simulink model "EPA_Walker"  (R2018a)
settings: Solver=FixedStepDiscrete  StartTime=0.0  StopTime=inf  FixedStep=0.001  RelTol=1e-3  EnableMultiTasking=on
model workspace (MAT data in the model file):
  MCOS : class17 (value not decoded)
undefined symbols (not defined in the file or in its folder): bits_current, bits_GRF, bits_Kd, bits_Kp, bits_position, bits_velocity, deadzone_in_TIB, deadzone_out_TIB, GRF_MAX, GRF_MIN, k_p_TIB, KD_MAX, KD_MIN, KP_MAX, KP_MIN, P_MAX, P_MIN, PressureFilter_CutOffFreq, PressureFilter_Gain, ReadingVoltage, T_MAX, T_MIN, V_MAX, V_MIN, voltageBias_GAS, voltageBias_GL, voltageBias_HAM, voltageBias_IL, voltageBias_POP, voltageBias_RF, voltageBias_SOL, voltageBias_TIB, voltageBias_VAS, voltageMultiplier_GAS, voltageMultiplier_GL, voltageMultiplier_HAM, voltageMultiplier_IL, voltageMultiplier_POP, voltageMultiplier_RF, voltageMultiplier_SOL, voltageMultiplier_TIB, voltageMultiplier_VAS, VoltageResolution
libraries: xpcethercatlib x139, simulink x19, peGeneralControl x18, slrtlib x9
(part 2 of 5)

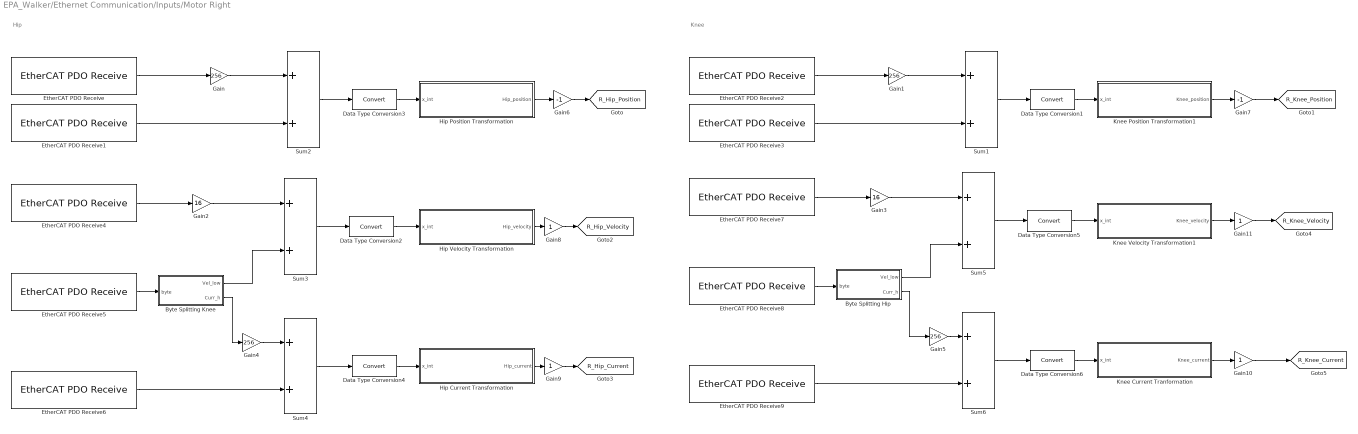
== system EPA_Walker/Ethernet Communication/Inputs/Motor Right ==
  note: Hip
  note: Knee
  Byte Splitting Hip : MATLAB Function  TreatAsAtomicUnit=on
  Byte Splitting Knee : MATLAB Function  TreatAsAtomicUnit=on
  Data Type Conversion{1..6} (6 alike) : DataTypeConversion
  EtherCAT PDO Receive : xpcethercatlib/EtherCAT PDO Receive  Priority=2  sig_name=Motors_R.Inputs.Byte0  sig_offset=256  sig_type=uint8  type_size=8  sig_dim=1  device_id=0  sample_time=0.001000
      settings: SourceProductName=Simulink Real-Time  SourceProductBaseCode=XP
  EtherCAT PDO Receive1 : xpcethercatlib/EtherCAT PDO Receive  Priority=2  sig_name=Motors_R.Inputs.Byte1  sig_offset=264  sig_type=uint8  type_size=8  sig_dim=1  device_id=0  sample_time=0.001000
      settings: SourceProductName=Simulink Real-Time  SourceProductBaseCode=XP
  EtherCAT PDO Receive2 : xpcethercatlib/EtherCAT PDO Receive  Priority=2  sig_name=Motors_R.Inputs.Byte5  sig_offset=296  sig_type=uint8  type_size=8  sig_dim=1  device_id=0  sample_time=0.001000
      settings: SourceProductName=Simulink Real-Time  SourceProductBaseCode=XP
  EtherCAT PDO Receive3 : xpcethercatlib/EtherCAT PDO Receive  Priority=2  sig_name=Motors_R.Inputs.Byte6  sig_offset=304  sig_type=uint8  type_size=8  sig_dim=1  device_id=0  sample_time=0.001000
      settings: SourceProductName=Simulink Real-Time  SourceProductBaseCode=XP
  EtherCAT PDO Receive4 : xpcethercatlib/EtherCAT PDO Receive  Priority=2  sig_name=Motors_R.Inputs.Byte2  sig_offset=272  sig_type=uint8  type_size=8  sig_dim=1  device_id=0  sample_time=0.001000
      settings: SourceProductName=Simulink Real-Time  SourceProductBaseCode=XP
  EtherCAT PDO Receive5 : xpcethercatlib/EtherCAT PDO Receive  Priority=2  sig_name=Motors_R.Inputs.Byte3  sig_offset=280  sig_type=uint8  type_size=8  sig_dim=1  device_id=0  sample_time=0.001000
      settings: SourceProductName=Simulink Real-Time  SourceProductBaseCode=XP
  EtherCAT PDO Receive6 : xpcethercatlib/EtherCAT PDO Receive  Priority=2  sig_name=Motors_R.Inputs.Byte4  sig_offset=288  sig_type=uint8  type_size=8  sig_dim=1  device_id=0  sample_time=0.001000
      settings: SourceProductName=Simulink Real-Time  SourceProductBaseCode=XP
  EtherCAT PDO Receive7 : xpcethercatlib/EtherCAT PDO Receive  Priority=2  sig_name=Motors_R.Inputs.Byte7  sig_offset=312  sig_type=uint8  type_size=8  sig_dim=1  device_id=0  sample_time=0.001000
      settings: SourceProductName=Simulink Real-Time  SourceProductBaseCode=XP
  EtherCAT PDO Receive8 : xpcethercatlib/EtherCAT PDO Receive  Priority=2  sig_name=Motors_R.Inputs.Byte8  sig_offset=320  sig_type=uint8  type_size=8  sig_dim=1  device_id=0  sample_time=0.001000
      settings: SourceProductName=Simulink Real-Time  SourceProductBaseCode=XP
  EtherCAT PDO Receive9 : xpcethercatlib/EtherCAT PDO Receive  Priority=2  sig_name=Motors_R.Inputs.Byte9  sig_offset=328  sig_type=uint8  type_size=8  sig_dim=1  device_id=0  sample_time=0.001000
      settings: SourceProductName=Simulink Real-Time  SourceProductBaseCode=XP
  Gain{,1,4..5} (4 alike) : Gain  Gain=256
  Gain{8..11} (4 alike) : Gain
  Gain2 : Gain  Gain=16
  Gain3 : Gain  Gain=16
  Gain6 : Gain  Gain=-1
  Gain7 : Gain  Gain=-1
  Hip Current Transformation : MATLAB Function  TreatAsAtomicUnit=on
  Hip Position Transformation : MATLAB Function  TreatAsAtomicUnit=on
  Hip Velocity Transformation : MATLAB Function  TreatAsAtomicUnit=on
  Knee Current Tranformation : MATLAB Function  TreatAsAtomicUnit=on
  Knee Position Transformation1 : MATLAB Function  TreatAsAtomicUnit=on
  Knee Velocity Transformation1 : MATLAB Function  TreatAsAtomicUnit=on
  Sum{1..6} (6 alike) : Sum
  tag scope: R_Hip_Current=global, R_Hip_Position=global, R_Hip_Velocity=global, R_Knee_Current=global, R_Knee_Position=global, R_Knee_Velocity=global
  wires:
  EtherCAT PDO Receive/1 -> Gain/1
  Sum2/1 -> Data Type Conversion3/1
  Data Type Conversion3/1 -> Hip Position Transformation/1(x_int)
  Gain/1 -> Sum2/1
  EtherCAT PDO Receive1/1 -> Sum2/2
  EtherCAT PDO Receive3/1 -> Sum1/2
  Gain1/1 -> Sum1/1
  Data Type Conversion1/1 -> Knee Position Transformation1/1(x_int)
  EtherCAT PDO Receive2/1 -> Gain1/1
  Sum1/1 -> Data Type Conversion1/1
  EtherCAT PDO Receive5/1 -> Byte Splitting Knee/1(byte)
  EtherCAT PDO Receive4/1 -> Gain2/1
  Gain2/1 -> Sum3/1
  Byte Splitting Knee/1(Vel_low) -> Sum3/2
  EtherCAT PDO Receive6/1 -> Sum4/2
  Data Type Conversion2/1 -> Hip Velocity Transformation/1(x_int)
  Sum3/1 -> Data Type Conversion2/1
  Data Type Conversion4/1 -> Hip Current Transformation/1(x_int)
  Sum4/1 -> Data Type Conversion4/1
  EtherCAT PDO Receive7/1 -> Gain3/1
  Sum5/1 -> Data Type Conversion5/1
  Gain3/1 -> Sum5/1
  EtherCAT PDO Receive9/1 -> Sum6/2
  EtherCAT PDO Receive8/1 -> Byte Splitting Hip/1(byte)
  Byte Splitting Hip/2(Curr_h) -> Gain5/1
  Sum6/1 -> Data Type Conversion6/1
  Byte Splitting Hip/1(Vel_low) -> Sum5/2
  Hip Position Transformation/1(Hip_position) -> Gain6/1
  Hip Velocity Transformation/1(Hip_velocity) -> Gain8/1
  Hip Current Transformation/1(Hip_current) -> Gain9/1
  Knee Position Transformation1/1(Knee_position) -> Gain7/1
  Knee Velocity Transformation1/1(Knee_velocity) -> Gain11/1
  Data Type Conversion5/1 -> Knee Velocity Transformation1/1(x_int)
  Knee Current Tranformation/1(Knee_current) -> Gain10/1
  Data Type Conversion6/1 -> Knee Current Tranformation/1(x_int)
  Gain4/1 -> Sum4/1
  Byte Splitting Knee/2(Curr_h) -> Gain4/1
  Gain5/1 -> Sum6/1
  Gain6/1 -> [R_Hip_Position]
  Gain7/1 -> [R_Knee_Position]
  Gain8/1 -> [R_Hip_Velocity]
  Gain9/1 -> [R_Hip_Current]
  Gain10/1 -> [R_Knee_Current]
  Gain11/1 -> [R_Knee_Velocity]

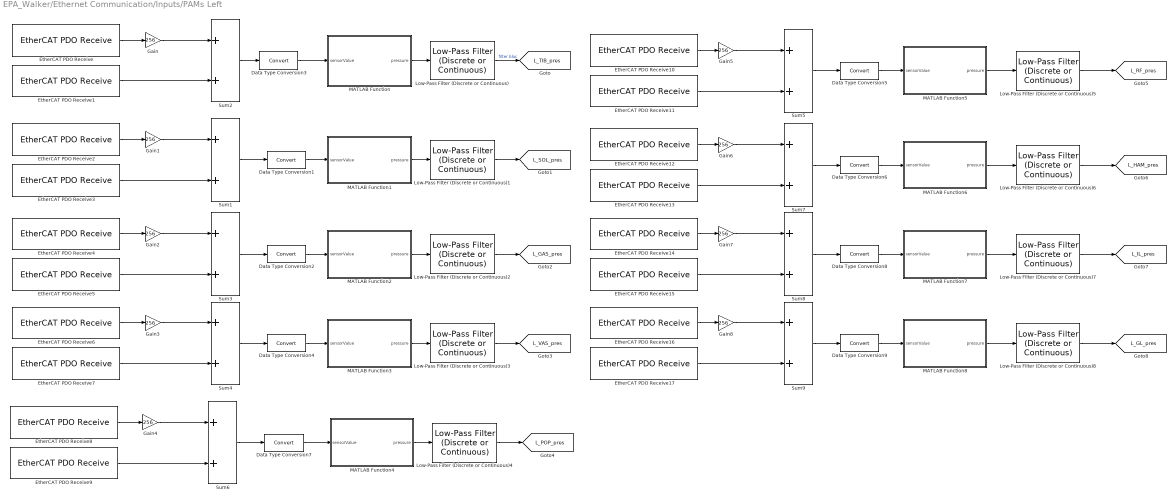
== system EPA_Walker/Ethernet Communication/Inputs/PAMs Left ==
  Data Type Conversion{1..9} (9 alike) : DataTypeConversion
  EtherCAT PDO Receive : xpcethercatlib/EtherCAT PDO Receive  Priority=2  sig_name=PAMs_L.Inputs.Byte0  sig_offset=1024  sig_type=uint8  type_size=8  sig_dim=1  device_id=0  sample_time=0.001000
      settings: SourceProductName=Simulink Real-Time  SourceProductBaseCode=XP
  EtherCAT PDO Receive1 : xpcethercatlib/EtherCAT PDO Receive  Priority=2  sig_name=PAMs_L.Inputs.Byte1  sig_offset=1032  sig_type=uint8  type_size=8  sig_dim=1  device_id=0  sample_time=0.001000
      settings: SourceProductName=Simulink Real-Time  SourceProductBaseCode=XP
  EtherCAT PDO Receive10 : xpcethercatlib/EtherCAT PDO Receive  Priority=2  sig_name=PAMs_L.Inputs.Byte10  sig_offset=1104  sig_type=uint8  type_size=8  sig_dim=1  device_id=0  sample_time=0.001000
      settings: SourceProductName=Simulink Real-Time  SourceProductBaseCode=XP
  EtherCAT PDO Receive11 : xpcethercatlib/EtherCAT PDO Receive  Priority=2  sig_name=PAMs_L.Inputs.Byte11  sig_offset=1112  sig_type=uint8  type_size=8  sig_dim=1  device_id=0  sample_time=0.001000
      settings: SourceProductName=Simulink Real-Time  SourceProductBaseCode=XP
  EtherCAT PDO Receive12 : xpcethercatlib/EtherCAT PDO Receive  Priority=2  sig_name=PAMs_L.Inputs.Byte12  sig_offset=1120  sig_type=uint8  type_size=8  sig_dim=1  device_id=0  sample_time=0.001000
      settings: SourceProductName=Simulink Real-Time  SourceProductBaseCode=XP
  EtherCAT PDO Receive13 : xpcethercatlib/EtherCAT PDO Receive  Priority=2  sig_name=PAMs_L.Inputs.Byte13  sig_offset=1128  sig_type=uint8  type_size=8  sig_dim=1  device_id=0  sample_time=0.001000
      settings: SourceProductName=Simulink Real-Time  SourceProductBaseCode=XP
  EtherCAT PDO Receive14 : xpcethercatlib/EtherCAT PDO Receive  Priority=2  sig_name=PAMs_L.Inputs.Byte14  sig_offset=1136  sig_type=uint8  type_size=8  sig_dim=1  device_id=0  sample_time=0.001000
      settings: SourceProductName=Simulink Real-Time  SourceProductBaseCode=XP
  EtherCAT PDO Receive15 : xpcethercatlib/EtherCAT PDO Receive  Priority=2  sig_name=PAMs_L.Inputs.Byte15  sig_offset=1144  sig_type=uint8  type_size=8  sig_dim=1  device_id=0  sample_time=0.001000
      settings: SourceProductName=Simulink Real-Time  SourceProductBaseCode=XP
  EtherCAT PDO Receive16 : xpcethercatlib/EtherCAT PDO Receive  Priority=2  sig_name=PAMs_L.Inputs.Byte16  sig_offset=1152  sig_type=uint8  type_size=8  sig_dim=1  device_id=0  sample_time=0.001000
      settings: SourceProductName=Simulink Real-Time  SourceProductBaseCode=XP
  EtherCAT PDO Receive17 : xpcethercatlib/EtherCAT PDO Receive  Priority=2  sig_name=PAMs_L.Inputs.Byte17  sig_offset=1160  sig_type=uint8  type_size=8  sig_dim=1  device_id=0  sample_time=0.001000
      settings: SourceProductName=Simulink Real-Time  SourceProductBaseCode=XP
  EtherCAT PDO Receive2 : xpcethercatlib/EtherCAT PDO Receive  Priority=2  sig_name=PAMs_L.Inputs.Byte2  sig_offset=1040  sig_type=uint8  type_size=8  sig_dim=1  device_id=0  sample_time=0.001000
      settings: SourceProductName=Simulink Real-Time  SourceProductBaseCode=XP
  EtherCAT PDO Receive3 : xpcethercatlib/EtherCAT PDO Receive  Priority=2  sig_name=PAMs_L.Inputs.Byte3  sig_offset=1048  sig_type=uint8  type_size=8  sig_dim=1  device_id=0  sample_time=0.001000
      settings: SourceProductName=Simulink Real-Time  SourceProductBaseCode=XP
  EtherCAT PDO Receive4 : xpcethercatlib/EtherCAT PDO Receive  Priority=2  sig_name=PAMs_L.Inputs.Byte4  sig_offset=1056  sig_type=uint8  type_size=8  sig_dim=1  device_id=0  sample_time=0.001000
      settings: SourceProductName=Simulink Real-Time  SourceProductBaseCode=XP
  EtherCAT PDO Receive5 : xpcethercatlib/EtherCAT PDO Receive  Priority=2  sig_name=PAMs_L.Inputs.Byte5  sig_offset=1064  sig_type=uint8  type_size=8  sig_dim=1  device_id=0  sample_time=0.001000
      settings: SourceProductName=Simulink Real-Time  SourceProductBaseCode=XP
  EtherCAT PDO Receive6 : xpcethercatlib/EtherCAT PDO Receive  Priority=2  sig_name=PAMs_L.Inputs.Byte6  sig_offset=1072  sig_type=uint8  type_size=8  sig_dim=1  device_id=0  sample_time=0.001000
      settings: SourceProductName=Simulink Real-Time  SourceProductBaseCode=XP
  EtherCAT PDO Receive7 : xpcethercatlib/EtherCAT PDO Receive  Priority=2  sig_name=PAMs_L.Inputs.Byte7  sig_offset=1080  sig_type=uint8  type_size=8  sig_dim=1  device_id=0  sample_time=0.001000
      settings: SourceProductName=Simulink Real-Time  SourceProductBaseCode=XP
  EtherCAT PDO Receive8 : xpcethercatlib/EtherCAT PDO Receive  Priority=2  sig_name=PAMs_L.Inputs.Byte8  sig_offset=1088  sig_type=uint8  type_size=8  sig_dim=1  device_id=0  sample_time=0.001000
      settings: SourceProductName=Simulink Real-Time  SourceProductBaseCode=XP
  EtherCAT PDO Receive9 : xpcethercatlib/EtherCAT PDO Receive  Priority=2  sig_name=PAMs_L.Inputs.Byte9  sig_offset=1096  sig_type=uint8  type_size=8  sig_dim=1  device_id=0  sample_time=0.001000
      settings: SourceProductName=Simulink Real-Time  SourceProductBaseCode=XP
  Gain{,1..8} (9 alike) : Gain  Gain=256
  Low-Pass Filter (Discrete or Continuous){,1..8} (9 alike) : peGeneralControl/Low-Pass Filter (Discrete or Continuous)  K=PressureFilter_Gain  T=1/PressureFilter_CutOffFreq  B=inf  A=-inf  Ts=-1
  MATLAB Function : MATLAB Function  TreatAsAtomicUnit=on
  MATLAB Function1 : MATLAB Function  TreatAsAtomicUnit=on
  MATLAB Function2 : MATLAB Function  TreatAsAtomicUnit=on
  MATLAB Function3 : MATLAB Function  TreatAsAtomicUnit=on
  MATLAB Function4 : MATLAB Function  TreatAsAtomicUnit=on
  MATLAB Function5 : MATLAB Function  TreatAsAtomicUnit=on
  MATLAB Function6 : MATLAB Function  TreatAsAtomicUnit=on
  MATLAB Function7 : MATLAB Function  TreatAsAtomicUnit=on
  MATLAB Function8 : MATLAB Function  TreatAsAtomicUnit=on
  Sum{1..9} (9 alike) : Sum
  tag scope: L_GAS_pres=global, L_GL_pres=global, L_HAM_pres=global, L_IL_pres=global, L_POP_pres=global, L_RF_pres=global, L_SOL_pres=global, L_TIB_pres=global, L_VAS_pres=global
  wires:
  EtherCAT PDO Receive1/1 -> Sum2/2
  Sum2/1 -> Data Type Conversion3/1
  EtherCAT PDO Receive/1 -> Gain/1
  Gain/1 -> Sum2/1
  Data Type Conversion3/1 -> MATLAB Function/1(sensorValue)
  Gain1/1 -> Sum1/1
  EtherCAT PDO Receive3/1 -> Sum1/2
  EtherCAT PDO Receive2/1 -> Gain1/1
  Data Type Conversion1/1 -> MATLAB Function1/1(sensorValue)
  Sum1/1 -> Data Type Conversion1/1
  Data Type Conversion2/1 -> MATLAB Function2/1(sensorValue)
  EtherCAT PDO Receive4/1 -> Gain2/1
  Gain2/1 -> Sum3/1
  Sum3/1 -> Data Type Conversion2/1
  EtherCAT PDO Receive5/1 -> Sum3/2
  Sum4/1 -> Data Type Conversion4/1
  Data Type Conversion4/1 -> MATLAB Function3/1(sensorValue)
  EtherCAT PDO Receive6/1 -> Gain3/1
  Gain3/1 -> Sum4/1
  EtherCAT PDO Receive7/1 -> Sum4/2
  Gain4/1 -> Sum6/1
  Sum6/1 -> Data Type Conversion7/1
  EtherCAT PDO Receive8/1 -> Gain4/1
  Data Type Conversion5/1 -> MATLAB Function5/1(sensorValue)
  EtherCAT PDO Receive10/1 -> Gain5/1
  Gain5/1 -> Sum5/1
  EtherCAT PDO Receive11/1 -> Sum5/2
  Data Type Conversion7/1 -> MATLAB Function4/1(sensorValue)
  EtherCAT PDO Receive15/1 -> Sum8/2
  Gain7/1 -> Sum8/1
  EtherCAT PDO Receive14/1 -> Gain7/1
  Data Type Conversion8/1 -> MATLAB Function7/1(sensorValue)
  Sum7/1 -> Data Type Conversion6/1
  Data Type Conversion6/1 -> MATLAB Function6/1(sensorValue)
  EtherCAT PDO Receive12/1 -> Gain6/1
  Sum5/1 -> Data Type Conversion5/1
  Sum8/1 -> Data Type Conversion8/1
  EtherCAT PDO Receive9/1 -> Sum6/2
  Gain6/1 -> Sum7/1
  EtherCAT PDO Receive13/1 -> Sum7/2
  MATLAB Function/1(pressure) -> Low-Pass Filter (Discrete or Continuous)/1
  MATLAB Function1/1(pressure) -> Low-Pass Filter (Discrete or Continuous)1/1
  MATLAB Function2/1(pressure) -> Low-Pass Filter (Discrete or Continuous)2/1
  MATLAB Function3/1(pressure) -> Low-Pass Filter (Discrete or Continuous)3/1
  MATLAB Function4/1(pressure) -> Low-Pass Filter (Discrete or Continuous)4/1
  MATLAB Function5/1(pressure) -> Low-Pass Filter (Discrete or Continuous)5/1
  MATLAB Function6/1(pressure) -> Low-Pass Filter (Discrete or Continuous)6/1
  MATLAB Function7/1(pressure) -> Low-Pass Filter (Discrete or Continuous)7/1
  Sum9/1 -> Data Type Conversion9/1
  EtherCAT PDO Receive16/1 -> Gain8/1
  Data Type Conversion9/1 -> MATLAB Function8/1(sensorValue)
  Gain8/1 -> Sum9/1
  MATLAB Function8/1(pressure) -> Low-Pass Filter (Discrete or Continuous)8/1
  EtherCAT PDO Receive17/1 -> Sum9/2
  Low-Pass Filter (Discrete or Continuous)/1 -> [L_TIB_pres]  "filter bloc"
  Low-Pass Filter (Discrete or Continuous)1/1 -> [L_SOL_pres]
  Low-Pass Filter (Discrete or Continuous)2/1 -> [L_GAS_pres]
  Low-Pass Filter (Discrete or Continuous)3/1 -> [L_VAS_pres]
  Low-Pass Filter (Discrete or Continuous)4/1 -> [L_POP_pres]
  Low-Pass Filter (Discrete or Continuous)5/1 -> [L_RF_pres]
  Low-Pass Filter (Discrete or Continuous)6/1 -> [L_HAM_pres]
  Low-Pass Filter (Discrete or Continuous)7/1 -> [L_IL_pres]
  Low-Pass Filter (Discrete or Continuous)8/1 -> [L_GL_pres]

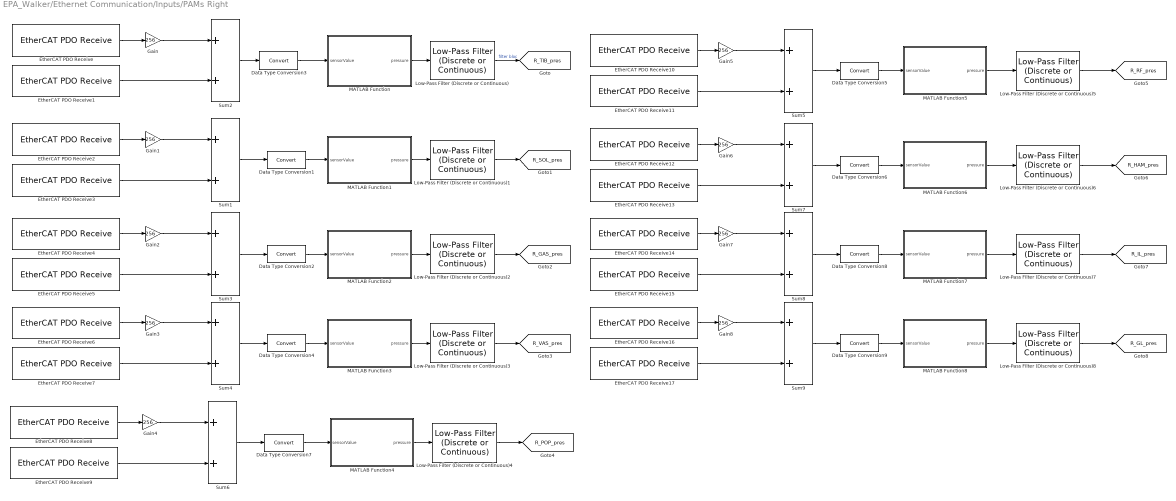
== system EPA_Walker/Ethernet Communication/Inputs/PAMs Right ==
  Data Type Conversion{1..9} (9 alike) : DataTypeConversion
  EtherCAT PDO Receive : xpcethercatlib/EtherCAT PDO Receive  Priority=2  sig_name=PAMs_R.Inputs.Byte0  sig_offset=512  sig_type=uint8  type_size=8  sig_dim=1  device_id=0  sample_time=0.001000
      settings: SourceProductName=Simulink Real-Time  SourceProductBaseCode=XP
  EtherCAT PDO Receive1 : xpcethercatlib/EtherCAT PDO Receive  Priority=2  sig_name=PAMs_R.Inputs.Byte1  sig_offset=520  sig_type=uint8  type_size=8  sig_dim=1  device_id=0  sample_time=0.001000
      settings: SourceProductName=Simulink Real-Time  SourceProductBaseCode=XP
  EtherCAT PDO Receive10 : xpcethercatlib/EtherCAT PDO Receive  Priority=2  sig_name=PAMs_R.Inputs.Byte10  sig_offset=592  sig_type=uint8  type_size=8  sig_dim=1  device_id=0  sample_time=0.001000
      settings: SourceProductName=Simulink Real-Time  SourceProductBaseCode=XP
  EtherCAT PDO Receive11 : xpcethercatlib/EtherCAT PDO Receive  Priority=2  sig_name=PAMs_R.Inputs.Byte11  sig_offset=600  sig_type=uint8  type_size=8  sig_dim=1  device_id=0  sample_time=0.001000
      settings: SourceProductName=Simulink Real-Time  SourceProductBaseCode=XP
  EtherCAT PDO Receive12 : xpcethercatlib/EtherCAT PDO Receive  Priority=2  sig_name=PAMs_R.Inputs.Byte12  sig_offset=608  sig_type=uint8  type_size=8  sig_dim=1  device_id=0  sample_time=0.001000
      settings: SourceProductName=Simulink Real-Time  SourceProductBaseCode=XP
  EtherCAT PDO Receive13 : xpcethercatlib/EtherCAT PDO Receive  Priority=2  sig_name=PAMs_R.Inputs.Byte13  sig_offset=616  sig_type=uint8  type_size=8  sig_dim=1  device_id=0  sample_time=0.001000
      settings: SourceProductName=Simulink Real-Time  SourceProductBaseCode=XP
  EtherCAT PDO Receive14 : xpcethercatlib/EtherCAT PDO Receive  Priority=2  sig_name=PAMs_R.Inputs.Byte14  sig_offset=624  sig_type=uint8  type_size=8  sig_dim=1  device_id=0  sample_time=0.001000
      settings: SourceProductName=Simulink Real-Time  SourceProductBaseCode=XP
  EtherCAT PDO Receive15 : xpcethercatlib/EtherCAT PDO Receive  Priority=2  sig_name=PAMs_R.Inputs.Byte15  sig_offset=632  sig_type=uint8  type_size=8  sig_dim=1  device_id=0  sample_time=0.001000
      settings: SourceProductName=Simulink Real-Time  SourceProductBaseCode=XP
  EtherCAT PDO Receive16 : xpcethercatlib/EtherCAT PDO Receive  Priority=2  sig_name=PAMs_R.Inputs.Byte16  sig_offset=640  sig_type=uint8  type_size=8  sig_dim=1  device_id=0  sample_time=0.001000
      settings: SourceProductName=Simulink Real-Time  SourceProductBaseCode=XP
  EtherCAT PDO Receive17 : xpcethercatlib/EtherCAT PDO Receive  Priority=2  sig_name=PAMs_R.Inputs.Byte17  sig_offset=648  sig_type=uint8  type_size=8  sig_dim=1  device_id=0  sample_time=0.001000
      settings: SourceProductName=Simulink Real-Time  SourceProductBaseCode=XP
  EtherCAT PDO Receive2 : xpcethercatlib/EtherCAT PDO Receive  Priority=2  sig_name=PAMs_R.Inputs.Byte2  sig_offset=528  sig_type=uint8  type_size=8  sig_dim=1  device_id=0  sample_time=0.001000
      settings: SourceProductName=Simulink Real-Time  SourceProductBaseCode=XP
  EtherCAT PDO Receive3 : xpcethercatlib/EtherCAT PDO Receive  Priority=2  sig_name=PAMs_R.Inputs.Byte3  sig_offset=536  sig_type=uint8  type_size=8  sig_dim=1  device_id=0  sample_time=0.001000
      settings: SourceProductName=Simulink Real-Time  SourceProductBaseCode=XP
  EtherCAT PDO Receive4 : xpcethercatlib/EtherCAT PDO Receive  Priority=2  sig_name=PAMs_R.Inputs.Byte4  sig_offset=544  sig_type=uint8  type_size=8  sig_dim=1  device_id=0  sample_time=0.001000
      settings: SourceProductName=Simulink Real-Time  SourceProductBaseCode=XP
  EtherCAT PDO Receive5 : xpcethercatlib/EtherCAT PDO Receive  Priority=2  sig_name=PAMs_R.Inputs.Byte5  sig_offset=552  sig_type=uint8  type_size=8  sig_dim=1  device_id=0  sample_time=0.001000
      settings: SourceProductName=Simulink Real-Time  SourceProductBaseCode=XP
  EtherCAT PDO Receive6 : xpcethercatlib/EtherCAT PDO Receive  Priority=2  sig_name=PAMs_R.Inputs.Byte6  sig_offset=560  sig_type=uint8  type_size=8  sig_dim=1  device_id=0  sample_time=0.001000
      settings: SourceProductName=Simulink Real-Time  SourceProductBaseCode=XP
  EtherCAT PDO Receive7 : xpcethercatlib/EtherCAT PDO Receive  Priority=2  sig_name=PAMs_R.Inputs.Byte7  sig_offset=568  sig_type=uint8  type_size=8  sig_dim=1  device_id=0  sample_time=0.001000
      settings: SourceProductName=Simulink Real-Time  SourceProductBaseCode=XP
  EtherCAT PDO Receive8 : xpcethercatlib/EtherCAT PDO Receive  Priority=2  sig_name=PAMs_R.Inputs.Byte8  sig_offset=576  sig_type=uint8  type_size=8  sig_dim=1  device_id=0  sample_time=0.001000
      settings: SourceProductName=Simulink Real-Time  SourceProductBaseCode=XP
  EtherCAT PDO Receive9 : xpcethercatlib/EtherCAT PDO Receive  Priority=2  sig_name=PAMs_R.Inputs.Byte9  sig_offset=584  sig_type=uint8  type_size=8  sig_dim=1  device_id=0  sample_time=0.001000
      settings: SourceProductName=Simulink Real-Time  SourceProductBaseCode=XP
  Gain{,1..8} (9 alike) : Gain  Gain=256
  Low-Pass Filter (Discrete or Continuous){,1..8} (9 alike) : peGeneralControl/Low-Pass Filter (Discrete or Continuous)  K=PressureFilter_Gain  T=1/PressureFilter_CutOffFreq  B=inf  A=-inf  Ts=-1
  MATLAB Function : MATLAB Function  TreatAsAtomicUnit=on
  MATLAB Function1 : MATLAB Function  TreatAsAtomicUnit=on
  MATLAB Function2 : MATLAB Function  TreatAsAtomicUnit=on
  MATLAB Function3 : MATLAB Function  TreatAsAtomicUnit=on
  MATLAB Function4 : MATLAB Function  TreatAsAtomicUnit=on
  MATLAB Function5 : MATLAB Function  TreatAsAtomicUnit=on
  MATLAB Function6 : MATLAB Function  TreatAsAtomicUnit=on
  MATLAB Function7 : MATLAB Function  TreatAsAtomicUnit=on
  MATLAB Function8 : MATLAB Function  TreatAsAtomicUnit=on
  Sum{1..9} (9 alike) : Sum
  tag scope: R_GAS_pres=global, R_GL_pres=global, R_HAM_pres=global, R_IL_pres=global, R_POP_pres=global, R_RF_pres=global, R_SOL_pres=global, R_TIB_pres=global, R_VAS_pres=global
  wires:
  EtherCAT PDO Receive1/1 -> Sum2/2
  Sum2/1 -> Data Type Conversion3/1
  EtherCAT PDO Receive/1 -> Gain/1
  Gain/1 -> Sum2/1
  Data Type Conversion3/1 -> MATLAB Function/1(sensorValue)
  Gain1/1 -> Sum1/1
  EtherCAT PDO Receive3/1 -> Sum1/2
  EtherCAT PDO Receive2/1 -> Gain1/1
  Data Type Conversion1/1 -> MATLAB Function1/1(sensorValue)
  Sum1/1 -> Data Type Conversion1/1
  Data Type Conversion2/1 -> MATLAB Function2/1(sensorValue)
  EtherCAT PDO Receive4/1 -> Gain2/1
  Gain2/1 -> Sum3/1
  Sum3/1 -> Data Type Conversion2/1
  EtherCAT PDO Receive5/1 -> Sum3/2
  Sum4/1 -> Data Type Conversion4/1
  Data Type Conversion4/1 -> MATLAB Function3/1(sensorValue)
  EtherCAT PDO Receive6/1 -> Gain3/1
  Gain3/1 -> Sum4/1
  EtherCAT PDO Receive7/1 -> Sum4/2
  Gain4/1 -> Sum6/1
  Sum6/1 -> Data Type Conversion7/1
  EtherCAT PDO Receive8/1 -> Gain4/1
  Data Type Conversion5/1 -> MATLAB Function5/1(sensorValue)
  EtherCAT PDO Receive10/1 -> Gain5/1
  Gain5/1 -> Sum5/1
  EtherCAT PDO Receive11/1 -> Sum5/2
  Data Type Conversion7/1 -> MATLAB Function4/1(sensorValue)
  EtherCAT PDO Receive15/1 -> Sum8/2
  Gain7/1 -> Sum8/1
  EtherCAT PDO Receive14/1 -> Gain7/1
  Data Type Conversion8/1 -> MATLAB Function7/1(sensorValue)
  Sum7/1 -> Data Type Conversion6/1
  Data Type Conversion6/1 -> MATLAB Function6/1(sensorValue)
  EtherCAT PDO Receive12/1 -> Gain6/1
  Sum5/1 -> Data Type Conversion5/1
  Sum8/1 -> Data Type Conversion8/1
  EtherCAT PDO Receive9/1 -> Sum6/2
  Gain6/1 -> Sum7/1
  EtherCAT PDO Receive13/1 -> Sum7/2
  MATLAB Function/1(pressure) -> Low-Pass Filter (Discrete or Continuous)/1
  MATLAB Function1/1(pressure) -> Low-Pass Filter (Discrete or Continuous)1/1
  MATLAB Function2/1(pressure) -> Low-Pass Filter (Discrete or Continuous)2/1
  MATLAB Function3/1(pressure) -> Low-Pass Filter (Discrete or Continuous)3/1
  MATLAB Function4/1(pressure) -> Low-Pass Filter (Discrete or Continuous)4/1
  MATLAB Function5/1(pressure) -> Low-Pass Filter (Discrete or Continuous)5/1
  MATLAB Function6/1(pressure) -> Low-Pass Filter (Discrete or Continuous)6/1
  MATLAB Function7/1(pressure) -> Low-Pass Filter (Discrete or Continuous)7/1
  Sum9/1 -> Data Type Conversion9/1
  EtherCAT PDO Receive16/1 -> Gain8/1
  Data Type Conversion9/1 -> MATLAB Function8/1(sensorValue)
  Gain8/1 -> Sum9/1
  MATLAB Function8/1(pressure) -> Low-Pass Filter (Discrete or Continuous)8/1
  EtherCAT PDO Receive17/1 -> Sum9/2
  Low-Pass Filter (Discrete or Continuous)/1 -> [R_TIB_pres]  "filter bloc"
  Low-Pass Filter (Discrete or Continuous)1/1 -> [R_SOL_pres]
  Low-Pass Filter (Discrete or Continuous)2/1 -> [R_GAS_pres]
  Low-Pass Filter (Discrete or Continuous)3/1 -> [R_VAS_pres]
  Low-Pass Filter (Discrete or Continuous)4/1 -> [R_POP_pres]
  Low-Pass Filter (Discrete or Continuous)5/1 -> [R_RF_pres]
  Low-Pass Filter (Discrete or Continuous)6/1 -> [R_HAM_pres]
  Low-Pass Filter (Discrete or Continuous)7/1 -> [R_IL_pres]
  Low-Pass Filter (Discrete or Continuous)8/1 -> [R_GL_pres]

== system EPA_Walker/Ethernet Communication/Outputs/GRF Slave ==
  Data Type Conversion13 : DataTypeConversion
  EtherCAT PDO Transmit 2 : xpcethercatlib/EtherCAT PDO Transmit   Priority=3  sig_name=GRF.Outputs.Byte0  sig_offset=0  sig_type=uint8  type_size=8  sig_dim=1  device_id=0  sample_time=0.001000
      settings: SourceProductName=Simulink Real-Time  SourceProductBaseCode=XP
  wires:
  Data Type Conversion13/1 -> EtherCAT PDO Transmit 2/1
  [GRF_Operation_Mode] -> Data Type Conversion13/1

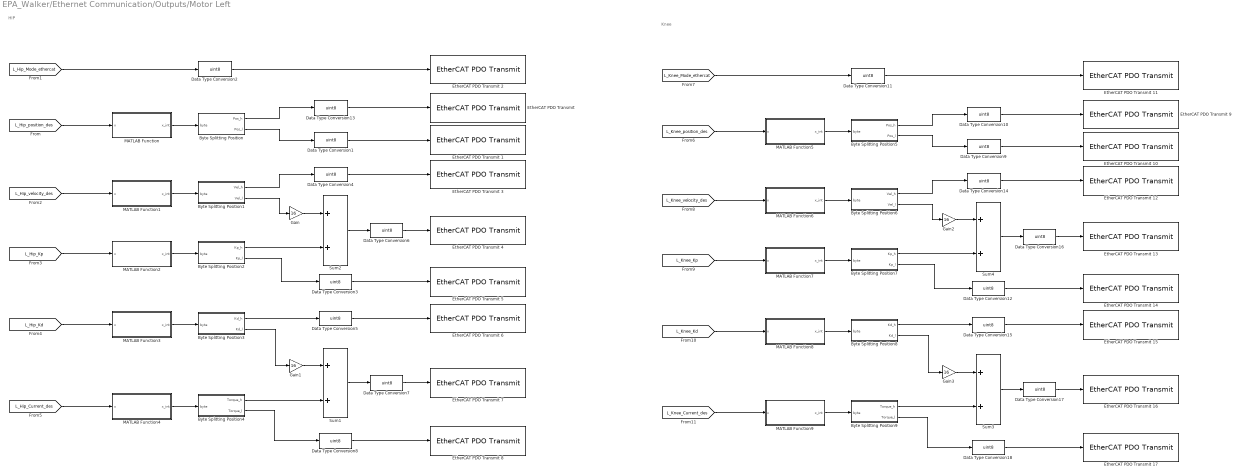
== system EPA_Walker/Ethernet Communication/Outputs/Motor Left ==
  note: HIP
  note: Knee
  Byte Splitting Position : MATLAB Function  TreatAsAtomicUnit=on
  Byte Splitting Position1 : MATLAB Function  TreatAsAtomicUnit=on
  Byte Splitting Position2 : MATLAB Function  TreatAsAtomicUnit=on
  Byte Splitting Position3 : MATLAB Function  TreatAsAtomicUnit=on
  Byte Splitting Position4 : MATLAB Function  TreatAsAtomicUnit=on
  Byte Splitting Position5 : MATLAB Function  TreatAsAtomicUnit=on
  Byte Splitting Position6 : MATLAB Function  TreatAsAtomicUnit=on
  Byte Splitting Position7 : MATLAB Function  TreatAsAtomicUnit=on
  Byte Splitting Position8 : MATLAB Function  TreatAsAtomicUnit=on
  Byte Splitting Position9 : MATLAB Function  TreatAsAtomicUnit=on
  Data Type Conversion{1,3..18} (17 alike) : DataTypeConversion  OutDataTypeStr=uint8
  Data Type Conversion2 : DataTypeConversion  OutDataTypeStr=uint8  RndMeth=Ceiling
  "EtherCAT PDO Transmit " : xpcethercatlib/EtherCAT PDO Transmit   Priority=3  sig_name=Motors_L.Outputs.Byte1  sig_offset=776  sig_type=uint8  type_size=8  sig_dim=1  device_id=0  sample_time=0.001000
      settings: SourceProductName=Simulink Real-Time  SourceProductBaseCode=XP
  EtherCAT PDO Transmit 1 : xpcethercatlib/EtherCAT PDO Transmit   Priority=3  sig_name=Motors_L.Outputs.Byte2  sig_offset=784  sig_type=uint8  type_size=8  sig_dim=1  device_id=0  sample_time=0.001000
      settings: SourceProductName=Simulink Real-Time  SourceProductBaseCode=XP
  EtherCAT PDO Transmit 10 : xpcethercatlib/EtherCAT PDO Transmit   Priority=3  sig_name=Motors_L.Outputs.Byte11  sig_offset=856  sig_type=uint8  type_size=8  sig_dim=1  device_id=0  sample_time=0.001000
      settings: SourceProductName=Simulink Real-Time  SourceProductBaseCode=XP
  EtherCAT PDO Transmit 11 : xpcethercatlib/EtherCAT PDO Transmit   Priority=3  sig_name=Motors_L.Outputs.Byte9  sig_offset=840  sig_type=uint8  type_size=8  sig_dim=1  device_id=0  sample_time=0.001000
      settings: SourceProductName=Simulink Real-Time  SourceProductBaseCode=XP
  EtherCAT PDO Transmit 12 : xpcethercatlib/EtherCAT PDO Transmit   Priority=3  sig_name=Motors_L.Outputs.Byte12  sig_offset=864  sig_type=uint8  type_size=8  sig_dim=1  device_id=0  sample_time=0.001000
      settings: SourceProductName=Simulink Real-Time  SourceProductBaseCode=XP
  EtherCAT PDO Transmit 13 : xpcethercatlib/EtherCAT PDO Transmit   Priority=3  sig_name=Motors_L.Outputs.Byte13  sig_offset=872  sig_type=uint8  type_size=8  sig_dim=1  device_id=0  sample_time=0.001000
      settings: SourceProductName=Simulink Real-Time  SourceProductBaseCode=XP
  EtherCAT PDO Transmit 14 : xpcethercatlib/EtherCAT PDO Transmit   Priority=3  sig_name=Motors_L.Outputs.Byte14  sig_offset=880  sig_type=uint8  type_size=8  sig_dim=1  device_id=0  sample_time=0.001000
      settings: SourceProductName=Simulink Real-Time  SourceProductBaseCode=XP
  EtherCAT PDO Transmit 15 : xpcethercatlib/EtherCAT PDO Transmit   Priority=3  sig_name=Motors_L.Outputs.Byte15  sig_offset=888  sig_type=uint8  type_size=8  sig_dim=1  device_id=0  sample_time=0.001000
      settings: SourceProductName=Simulink Real-Time  SourceProductBaseCode=XP
  EtherCAT PDO Transmit 16 : xpcethercatlib/EtherCAT PDO Transmit   Priority=3  sig_name=Motors_L.Outputs.Byte16  sig_offset=896  sig_type=uint8  type_size=8  sig_dim=1  device_id=0  sample_time=0.001000
      settings: SourceProductName=Simulink Real-Time  SourceProductBaseCode=XP
  EtherCAT PDO Transmit 17 : xpcethercatlib/EtherCAT PDO Transmit   Priority=3  sig_name=Motors_L.Outputs.Byte17  sig_offset=904  sig_type=uint8  type_size=8  sig_dim=1  device_id=0  sample_time=0.001000
      settings: SourceProductName=Simulink Real-Time  SourceProductBaseCode=XP
  EtherCAT PDO Transmit 2 : xpcethercatlib/EtherCAT PDO Transmit   Priority=3  sig_name=Motors_L.Outputs.Byte0  sig_offset=768  sig_type=uint8  type_size=8  sig_dim=1  device_id=0  sample_time=0.001000
      settings: SourceProductName=Simulink Real-Time  SourceProductBaseCode=XP
  EtherCAT PDO Transmit 3 : xpcethercatlib/EtherCAT PDO Transmit   Priority=3  sig_name=Motors_L.Outputs.Byte3  sig_offset=792  sig_type=uint8  type_size=8  sig_dim=1  device_id=0  sample_time=0.001000
      settings: SourceProductName=Simulink Real-Time  SourceProductBaseCode=XP
  EtherCAT PDO Transmit 4 : xpcethercatlib/EtherCAT PDO Transmit   Priority=3  sig_name=Motors_L.Outputs.Byte4  sig_offset=800  sig_type=uint8  type_size=8  sig_dim=1  device_id=0  sample_time=0.001000
      settings: SourceProductName=Simulink Real-Time  SourceProductBaseCode=XP
  EtherCAT PDO Transmit 5 : xpcethercatlib/EtherCAT PDO Transmit   Priority=3  sig_name=Motors_L.Outputs.Byte5  sig_offset=808  sig_type=uint8  type_size=8  sig_dim=1  device_id=0  sample_time=0.001000
      settings: SourceProductName=Simulink Real-Time  SourceProductBaseCode=XP
  EtherCAT PDO Transmit 6 : xpcethercatlib/EtherCAT PDO Transmit   Priority=3  sig_name=Motors_L.Outputs.Byte6  sig_offset=816  sig_type=uint8  type_size=8  sig_dim=1  device_id=0  sample_time=0.001000
      settings: SourceProductName=Simulink Real-Time  SourceProductBaseCode=XP
  EtherCAT PDO Transmit 7 : xpcethercatlib/EtherCAT PDO Transmit   Priority=3  sig_name=Motors_L.Outputs.Byte7  sig_offset=824  sig_type=uint8  type_size=8  sig_dim=1  device_id=0  sample_time=0.001000
      settings: SourceProductName=Simulink Real-Time  SourceProductBaseCode=XP
  EtherCAT PDO Transmit 8 : xpcethercatlib/EtherCAT PDO Transmit   Priority=3  sig_name=Motors_L.Outputs.Byte8  sig_offset=832  sig_type=uint8  type_size=8  sig_dim=1  device_id=0  sample_time=0.001000
      settings: SourceProductName=Simulink Real-Time  SourceProductBaseCode=XP
  EtherCAT PDO Transmit 9 : xpcethercatlib/EtherCAT PDO Transmit   Priority=3  sig_name=Motors_L.Outputs.Byte10  sig_offset=848  sig_type=uint8  type_size=8  sig_dim=1  device_id=0  sample_time=0.001000
      settings: SourceProductName=Simulink Real-Time  SourceProductBaseCode=XP
  Gain{,1..3} (4 alike) : Gain  Gain=16
  MATLAB Function : MATLAB Function  TreatAsAtomicUnit=on
  MATLAB Function1 : MATLAB Function  TreatAsAtomicUnit=on
  MATLAB Function2 : MATLAB Function  TreatAsAtomicUnit=on
  MATLAB Function3 : MATLAB Function  TreatAsAtomicUnit=on
  MATLAB Function4 : MATLAB Function  TreatAsAtomicUnit=on
  MATLAB Function5 : MATLAB Function  TreatAsAtomicUnit=on
  MATLAB Function6 : MATLAB Function  TreatAsAtomicUnit=on
  MATLAB Function7 : MATLAB Function  TreatAsAtomicUnit=on
  MATLAB Function8 : MATLAB Function  TreatAsAtomicUnit=on
  MATLAB Function9 : MATLAB Function  TreatAsAtomicUnit=on
  Sum{1..4} (4 alike) : Sum
  wires:
  [L_Hip_position_des] -> MATLAB Function/1(x)
  MATLAB Function/1(x_int) -> Byte Splitting Position/1(byte)
  Byte Splitting Position/1(Pos_h) -> Data Type Conversion13/1
  Byte Splitting Position/2(Pos_l) -> Data Type Conversion1/1
  Data Type Conversion13/1 -> "EtherCAT PDO Transmit "/1
  Data Type Conversion1/1 -> EtherCAT PDO Transmit 1/1
  [L_Hip_Mode_ethercat] -> Data Type Conversion2/1
  Data Type Conversion2/1 -> EtherCAT PDO Transmit 2/1
  MATLAB Function1/1(x_int) -> Byte Splitting Position1/1(byte)
  Byte Splitting Position1/1(Vel_h) -> Data Type Conversion4/1
  Byte Splitting Position1/2(Vel_l) -> Gain/1
  [L_Hip_velocity_des] -> MATLAB Function1/1(x)
  Data Type Conversion4/1 -> EtherCAT PDO Transmit 3/1
  Gain/1 -> Sum2/1
  Sum2/1 -> Data Type Conversion6/1
  [L_Hip_Kp] -> MATLAB Function2/1(x)
  MATLAB Function2/1(x_int) -> Byte Splitting Position2/1(byte)
  Byte Splitting Position2/1(Kp_h) -> Sum2/2
  Data Type Conversion3/1 -> EtherCAT PDO Transmit 5/1
  Byte Splitting Position2/2(Kp_l) -> Data Type Conversion3/1
  [L_Hip_Kd] -> MATLAB Function3/1(x)
  MATLAB Function3/1(x_int) -> Byte Splitting Position3/1(byte)
  Byte Splitting Position3/2(Kd_l) -> Gain1/1
  Byte Splitting Position3/1(Kd_h) -> Data Type Conversion5/1
  Sum1/1 -> Data Type Conversion7/1
  Data Type Conversion5/1 -> EtherCAT PDO Transmit 6/1
  Gain1/1 -> Sum1/1
  Data Type Conversion6/1 -> EtherCAT PDO Transmit 4/1
  Data Type Conversion7/1 -> EtherCAT PDO Transmit 7/1
  [L_Hip_Current_des] -> MATLAB Function4/1(x)
  MATLAB Function4/1(x_int) -> Byte Splitting Position4/1(byte)
  Byte Splitting Position4/2(Torque_l) -> Data Type Conversion8/1
  Byte Splitting Position4/1(Torque_h) -> Sum1/2
  Data Type Conversion8/1 -> EtherCAT PDO Transmit 8/1
  Byte Splitting Position9/2(Torque_l) -> Data Type Conversion18/1
  Data Type Conversion15/1 -> EtherCAT PDO Transmit 15/1
  Byte Splitting Position8/2(Kd_l) -> Gain3/1
  Data Type Conversion17/1 -> EtherCAT PDO Transmit 16/1
  MATLAB Function5/1(x_int) -> Byte Splitting Position5/1(byte)
  Data Type Conversion10/1 -> EtherCAT PDO Transmit 9/1
  Data Type Conversion18/1 -> EtherCAT PDO Transmit 17/1
  MATLAB Function9/1(x_int) -> Byte Splitting Position9/1(byte)
  Byte Splitting Position9/1(Torque_h) -> Sum3/2
  [L_Knee_Mode_ethercat] -> Data Type Conversion11/1
  Data Type Conversion14/1 -> EtherCAT PDO Transmit 12/1
  [L_Knee_Kp] -> MATLAB Function7/1(x)
  MATLAB Function7/1(x_int) -> Byte Splitting Position7/1(byte)
  Byte Splitting Position7/2(Kp_l) -> Data Type Conversion12/1
  Byte Splitting Position8/1(Kd_h) -> Data Type Conversion15/1
  [L_Knee_Current_des] -> MATLAB Function9/1(x)
  Byte Splitting Position6/2(Vel_l) -> Gain2/1
  Data Type Conversion12/1 -> EtherCAT PDO Transmit 14/1
  Sum3/1 -> Data Type Conversion17/1
  Byte Splitting Position7/1(Kp_h) -> Sum4/2
  Byte Splitting Position5/2(Pos_l) -> Data Type Conversion9/1
  Data Type Conversion9/1 -> EtherCAT PDO Transmit 10/1
  Byte Splitting Position5/1(Pos_h) -> Data Type Conversion10/1
  Sum4/1 -> Data Type Conversion16/1
  Data Type Conversion11/1 -> EtherCAT PDO Transmit 11/1
  [L_Knee_velocity_des] -> MATLAB Function6/1(x)
  [L_Knee_position_des] -> MATLAB Function5/1(x)
  [L_Knee_Kd] -> MATLAB Function8/1(x)
  Gain2/1 -> Sum4/1
  Gain3/1 -> Sum3/1
  MATLAB Function8/1(x_int) -> Byte Splitting Position8/1(byte)
  Byte Splitting Position6/1(Vel_h) -> Data Type Conversion14/1
  MATLAB Function6/1(x_int) -> Byte Splitting Position6/1(byte)
  Data Type Conversion16/1 -> EtherCAT PDO Transmit 13/1

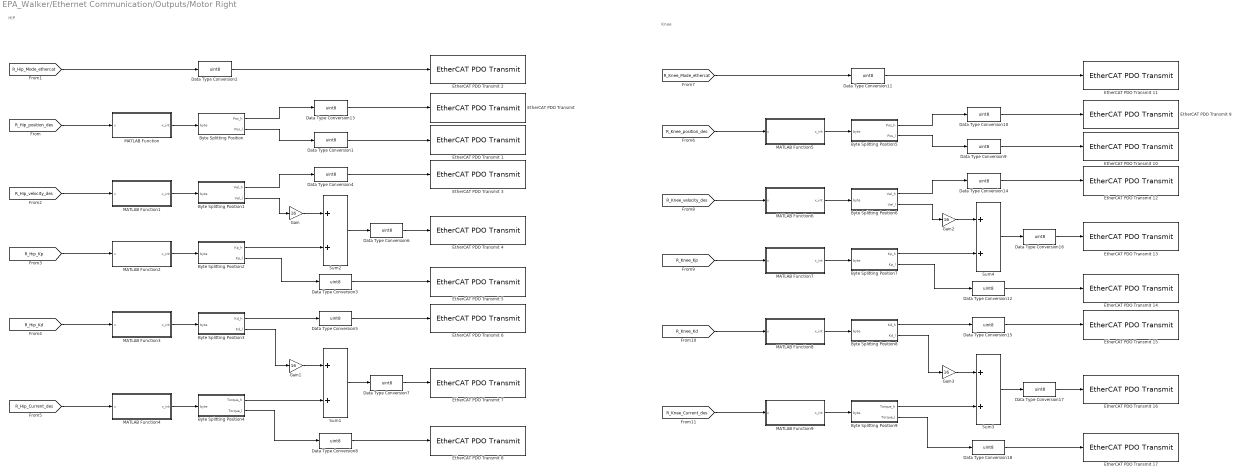
== system EPA_Walker/Ethernet Communication/Outputs/Motor Right ==
  note: HIP
  note: Knee
  Byte Splitting Position : MATLAB Function  TreatAsAtomicUnit=on
  Byte Splitting Position1 : MATLAB Function  TreatAsAtomicUnit=on
  Byte Splitting Position2 : MATLAB Function  TreatAsAtomicUnit=on
  Byte Splitting Position3 : MATLAB Function  TreatAsAtomicUnit=on
  Byte Splitting Position4 : MATLAB Function  TreatAsAtomicUnit=on
  Byte Splitting Position5 : MATLAB Function  TreatAsAtomicUnit=on
  Byte Splitting Position6 : MATLAB Function  TreatAsAtomicUnit=on
  Byte Splitting Position7 : MATLAB Function  TreatAsAtomicUnit=on
  Byte Splitting Position8 : MATLAB Function  TreatAsAtomicUnit=on
  Byte Splitting Position9 : MATLAB Function  TreatAsAtomicUnit=on
  Data Type Conversion{1,3..18} (17 alike) : DataTypeConversion  OutDataTypeStr=uint8
  Data Type Conversion2 : DataTypeConversion  OutDataTypeStr=uint8  RndMeth=Ceiling
  "EtherCAT PDO Transmit " : xpcethercatlib/EtherCAT PDO Transmit   Priority=3  sig_name=Motors_R.Outputs.Byte1  sig_offset=264  sig_type=uint8  type_size=8  sig_dim=1  device_id=0  sample_time=0.001000
      settings: SourceProductName=Simulink Real-Time  SourceProductBaseCode=XP
  EtherCAT PDO Transmit 1 : xpcethercatlib/EtherCAT PDO Transmit   Priority=3  sig_name=Motors_R.Outputs.Byte2  sig_offset=272  sig_type=uint8  type_size=8  sig_dim=1  device_id=0  sample_time=0.001000
      settings: SourceProductName=Simulink Real-Time  SourceProductBaseCode=XP
  EtherCAT PDO Transmit 10 : xpcethercatlib/EtherCAT PDO Transmit   Priority=3  sig_name=Motors_R.Outputs.Byte11  sig_offset=344  sig_type=uint8  type_size=8  sig_dim=1  device_id=0  sample_time=0.001000
      settings: SourceProductName=Simulink Real-Time  SourceProductBaseCode=XP
  EtherCAT PDO Transmit 11 : xpcethercatlib/EtherCAT PDO Transmit   Priority=3  sig_name=Motors_R.Outputs.Byte9  sig_offset=328  sig_type=uint8  type_size=8  sig_dim=1  device_id=0  sample_time=0.001000
      settings: SourceProductName=Simulink Real-Time  SourceProductBaseCode=XP
  EtherCAT PDO Transmit 12 : xpcethercatlib/EtherCAT PDO Transmit   Priority=3  sig_name=Motors_R.Outputs.Byte12  sig_offset=352  sig_type=uint8  type_size=8  sig_dim=1  device_id=0  sample_time=0.001000
      settings: SourceProductName=Simulink Real-Time  SourceProductBaseCode=XP
  EtherCAT PDO Transmit 13 : xpcethercatlib/EtherCAT PDO Transmit   Priority=3  sig_name=Motors_R.Outputs.Byte13  sig_offset=360  sig_type=uint8  type_size=8  sig_dim=1  device_id=0  sample_time=0.001000
      settings: SourceProductName=Simulink Real-Time  SourceProductBaseCode=XP
  EtherCAT PDO Transmit 14 : xpcethercatlib/EtherCAT PDO Transmit   Priority=3  sig_name=Motors_R.Outputs.Byte14  sig_offset=368  sig_type=uint8  type_size=8  sig_dim=1  device_id=0  sample_time=0.001000
      settings: SourceProductName=Simulink Real-Time  SourceProductBaseCode=XP
  EtherCAT PDO Transmit 15 : xpcethercatlib/EtherCAT PDO Transmit   Priority=3  sig_name=Motors_R.Outputs.Byte15  sig_offset=376  sig_type=uint8  type_size=8  sig_dim=1  device_id=0  sample_time=0.001000
      settings: SourceProductName=Simulink Real-Time  SourceProductBaseCode=XP
  EtherCAT PDO Transmit 16 : xpcethercatlib/EtherCAT PDO Transmit   Priority=3  sig_name=Motors_R.Outputs.Byte16  sig_offset=384  sig_type=uint8  type_size=8  sig_dim=1  device_id=0  sample_time=0.001000
      settings: SourceProductName=Simulink Real-Time  SourceProductBaseCode=XP
  EtherCAT PDO Transmit 17 : xpcethercatlib/EtherCAT PDO Transmit   Priority=3  sig_name=Motors_R.Outputs.Byte17  sig_offset=392  sig_type=uint8  type_size=8  sig_dim=1  device_id=0  sample_time=0.001000
      settings: SourceProductName=Simulink Real-Time  SourceProductBaseCode=XP
  EtherCAT PDO Transmit 2 : xpcethercatlib/EtherCAT PDO Transmit   Priority=3  sig_name=Motors_R.Outputs.Byte0  sig_offset=256  sig_type=uint8  type_size=8  sig_dim=1  device_id=0  sample_time=0.001000
      settings: SourceProductName=Simulink Real-Time  SourceProductBaseCode=XP
  EtherCAT PDO Transmit 3 : xpcethercatlib/EtherCAT PDO Transmit   Priority=3  sig_name=Motors_R.Outputs.Byte3  sig_offset=280  sig_type=uint8  type_size=8  sig_dim=1  device_id=0  sample_time=0.001000
      settings: SourceProductName=Simulink Real-Time  SourceProductBaseCode=XP
  EtherCAT PDO Transmit 4 : xpcethercatlib/EtherCAT PDO Transmit   Priority=3  sig_name=Motors_R.Outputs.Byte4  sig_offset=288  sig_type=uint8  type_size=8  sig_dim=1  device_id=0  sample_time=0.001000
      settings: SourceProductName=Simulink Real-Time  SourceProductBaseCode=XP
  EtherCAT PDO Transmit 5 : xpcethercatlib/EtherCAT PDO Transmit   Priority=3  sig_name=Motors_R.Outputs.Byte5  sig_offset=296  sig_type=uint8  type_size=8  sig_dim=1  device_id=0  sample_time=0.001000
      settings: SourceProductName=Simulink Real-Time  SourceProductBaseCode=XP
  EtherCAT PDO Transmit 6 : xpcethercatlib/EtherCAT PDO Transmit   Priority=3  sig_name=Motors_R.Outputs.Byte6  sig_offset=304  sig_type=uint8  type_size=8  sig_dim=1  device_id=0  sample_time=0.001000
      settings: SourceProductName=Simulink Real-Time  SourceProductBaseCode=XP
  EtherCAT PDO Transmit 7 : xpcethercatlib/EtherCAT PDO Transmit   Priority=3  sig_name=Motors_R.Outputs.Byte7  sig_offset=312  sig_type=uint8  type_size=8  sig_dim=1  device_id=0  sample_time=0.001000
      settings: SourceProductName=Simulink Real-Time  SourceProductBaseCode=XP
  EtherCAT PDO Transmit 8 : xpcethercatlib/EtherCAT PDO Transmit   Priority=3  sig_name=Motors_R.Outputs.Byte8  sig_offset=320  sig_type=uint8  type_size=8  sig_dim=1  device_id=0  sample_time=0.001000
      settings: SourceProductName=Simulink Real-Time  SourceProductBaseCode=XP
  EtherCAT PDO Transmit 9 : xpcethercatlib/EtherCAT PDO Transmit   Priority=3  sig_name=Motors_R.Outputs.Byte10  sig_offset=336  sig_type=uint8  type_size=8  sig_dim=1  device_id=0  sample_time=0.001000
      settings: SourceProductName=Simulink Real-Time  SourceProductBaseCode=XP
  Gain{,1..3} (4 alike) : Gain  Gain=16
  MATLAB Function : MATLAB Function  TreatAsAtomicUnit=on
  MATLAB Function1 : MATLAB Function  TreatAsAtomicUnit=on
  MATLAB Function2 : MATLAB Function  TreatAsAtomicUnit=on
  MATLAB Function3 : MATLAB Function  TreatAsAtomicUnit=on
  MATLAB Function4 : MATLAB Function  TreatAsAtomicUnit=on
  MATLAB Function5 : MATLAB Function  TreatAsAtomicUnit=on
  MATLAB Function6 : MATLAB Function  TreatAsAtomicUnit=on
  MATLAB Function7 : MATLAB Function  TreatAsAtomicUnit=on
  MATLAB Function8 : MATLAB Function  TreatAsAtomicUnit=on
  MATLAB Function9 : MATLAB Function  TreatAsAtomicUnit=on
  Sum{1..4} (4 alike) : Sum
  wires:
  [R_Hip_position_des] -> MATLAB Function/1(x)
  MATLAB Function/1(x_int) -> Byte Splitting Position/1(byte)
  Byte Splitting Position/1(Pos_h) -> Data Type Conversion13/1
  Byte Splitting Position/2(Pos_l) -> Data Type Conversion1/1
  Data Type Conversion13/1 -> "EtherCAT PDO Transmit "/1
  Data Type Conversion1/1 -> EtherCAT PDO Transmit 1/1
  [R_Hip_Mode_ethercat] -> Data Type Conversion2/1
  Data Type Conversion2/1 -> EtherCAT PDO Transmit 2/1
  MATLAB Function1/1(x_int) -> Byte Splitting Position1/1(byte)
  Byte Splitting Position1/1(Vel_h) -> Data Type Conversion4/1
  Byte Splitting Position1/2(Vel_l) -> Gain/1
  [R_Hip_velocity_des] -> MATLAB Function1/1(x)
  Data Type Conversion4/1 -> EtherCAT PDO Transmit 3/1
  Gain/1 -> Sum2/1
  Sum2/1 -> Data Type Conversion6/1
  [R_Hip_Kp] -> MATLAB Function2/1(x)
  MATLAB Function2/1(x_int) -> Byte Splitting Position2/1(byte)
  Byte Splitting Position2/1(Kp_h) -> Sum2/2
  Data Type Conversion3/1 -> EtherCAT PDO Transmit 5/1
  Byte Splitting Position2/2(Kp_l) -> Data Type Conversion3/1
  [R_Hip_Kd] -> MATLAB Function3/1(x)
  MATLAB Function3/1(x_int) -> Byte Splitting Position3/1(byte)
  Byte Splitting Position3/2(Kd_l) -> Gain1/1
  Byte Splitting Position3/1(Kd_h) -> Data Type Conversion5/1
  Sum1/1 -> Data Type Conversion7/1
  Data Type Conversion5/1 -> EtherCAT PDO Transmit 6/1
  Gain1/1 -> Sum1/1
  Data Type Conversion6/1 -> EtherCAT PDO Transmit 4/1
  Data Type Conversion7/1 -> EtherCAT PDO Transmit 7/1
  [R_Hip_Current_des] -> MATLAB Function4/1(x)
  MATLAB Function4/1(x_int) -> Byte Splitting Position4/1(byte)
  Byte Splitting Position4/2(Torque_l) -> Data Type Conversion8/1
  Byte Splitting Position4/1(Torque_h) -> Sum1/2
  Data Type Conversion8/1 -> EtherCAT PDO Transmit 8/1
  Byte Splitting Position9/2(Torque_l) -> Data Type Conversion18/1
  Data Type Conversion15/1 -> EtherCAT PDO Transmit 15/1
  Byte Splitting Position8/2(Kd_l) -> Gain3/1
  Data Type Conversion17/1 -> EtherCAT PDO Transmit 16/1
  MATLAB Function5/1(x_int) -> Byte Splitting Position5/1(byte)
  Data Type Conversion10/1 -> EtherCAT PDO Transmit 9/1
  Data Type Conversion18/1 -> EtherCAT PDO Transmit 17/1
  MATLAB Function9/1(x_int) -> Byte Splitting Position9/1(byte)
  Byte Splitting Position9/1(Torque_h) -> Sum3/2
  [R_Knee_Mode_ethercat] -> Data Type Conversion11/1
  Data Type Conversion14/1 -> EtherCAT PDO Transmit 12/1
  [R_Knee_Kp] -> MATLAB Function7/1(x)
  MATLAB Function7/1(x_int) -> Byte Splitting Position7/1(byte)
  Byte Splitting Position7/2(Kp_l) -> Data Type Conversion12/1
  Byte Splitting Position8/1(Kd_h) -> Data Type Conversion15/1
  [R_Knee_Current_des] -> MATLAB Function9/1(x)
  Byte Splitting Position6/2(Vel_l) -> Gain2/1
  Data Type Conversion12/1 -> EtherCAT PDO Transmit 14/1
  Sum3/1 -> Data Type Conversion17/1
  Byte Splitting Position7/1(Kp_h) -> Sum4/2
  Byte Splitting Position5/2(Pos_l) -> Data Type Conversion9/1
  Data Type Conversion9/1 -> EtherCAT PDO Transmit 10/1
  Byte Splitting Position5/1(Pos_h) -> Data Type Conversion10/1
  Sum4/1 -> Data Type Conversion16/1
  Data Type Conversion11/1 -> EtherCAT PDO Transmit 11/1
  [R_Knee_velocity_des] -> MATLAB Function6/1(x)
  [R_Knee_position_des] -> MATLAB Function5/1(x)
  [R_Knee_Kd] -> MATLAB Function8/1(x)
  Gain2/1 -> Sum4/1
  Gain3/1 -> Sum3/1
  MATLAB Function8/1(x_int) -> Byte Splitting Position8/1(byte)
  Byte Splitting Position6/1(Vel_h) -> Data Type Conversion14/1
  MATLAB Function6/1(x_int) -> Byte Splitting Position6/1(byte)
  Data Type Conversion16/1 -> EtherCAT PDO Transmit 13/1
